simulink model "ref_subsystem_test"  (Simulink 8.4)
settings: Solver=ode45  StartTime=0.0  StopTime=10.0  RelTol=1e-3
settings Model: Creator=arnaud  LastModifiedBy=arnaud
settings DataIOCC: SaveFormat=Structure  SignalLoggingSaveFormat=Dataset  SaveOutput=off  SaveTime=off
settings OptimizationCC: ExpressionDepthLimit=128
settings DebuggingCC: UnderspecifiedInitializationDetection=Simplified  MergeDetectMultiDrivingBlocksExec=error  FcnCallInpInsideContextMsg=EnableAllAsError  StateNameClashWarn=none
settings GRTTargetCC: CombineOutputUpdateFcns=on  GRTInterface=off

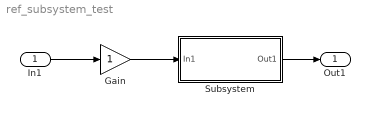
== system ref_subsystem_test ==
  In1 : Inport  OutDataTypeStr=double  PortDimensions=1  SampleTime=0
  Gain : Gain
  Subsystem : Subsystem  TreatAsAtomicUnit=on
  Out1 : Outport  OutDataTypeStr=double  PortDimensions=1  SampleTime=0
  wires:
  In1/1 -> Gain/1
  Subsystem/1(Out1) -> Out1/1
  Gain/1 -> Subsystem/1(In1)

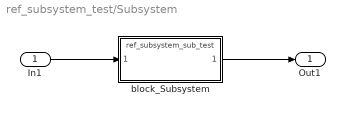
== system ref_subsystem_test/Subsystem ==
  In1 : Inport
  block_Subsystem : ModelReference  ModelNameDialog=ref_subsystem_sub_test.mdl  SimulationMode=Normal  ModelReferenceVersion=1.11  CopyOfModelName=ref_subsystem_sub_test.mdl  DefaultDataLogging=on
  Out1 : Outport
  wires:
  In1/1 -> block_Subsystem/1
  block_Subsystem/1 -> Out1/1
